simulink model "Auto_microgrid_forecasting_020822"  (R2020a)
settings: Solver=VariableStepAuto  StartTime=0.0  StopTime=50  MaxStep=1e-4  RelTol=1e-3
PreLoadFcn:
  | %run('FC_microgrid_param.m')
  | %load('gen_grid_init.mat')
InitFcn:
  | %load myisoModel_init;
  | run('FC_microgrid_param.m')
  | tic
  | run('CARTinitFcn.m')
  | %caseNo = 2;
  | 
  | %if (caseNo == 1)
  | %set_param(['Isolated_grid_paper_model_022521/SignalGen'], 'ActiveScenario', 'PStep222kW');
  | %else
  | %set_param(['Isolated_grid_paper_model_022521/SignalGen'], 'ActiveScenario', 'QStep222kVAr');
  | 
  | %end;
StopFcn:
  | toc
undefined symbols (not defined in the file or in its folder): breakpoints1, breakpoints2, cc_kp, cp_table_data, ctrl, D1, Delta, DiscIntNeverNeededParam, DT, FC_BESS, FC_PV_FirstSolar, find_system, Fnom, gcbh, libFC_BESS, libFC_PV, LowerLimit, magnitude, oversize, pll_ki, pll_kp, pq_ts, SOC_target, sps_rtmsupport, timer, Ts, ts, Ts_APC, Ts_Control, Ts_Power, UpperLimit
libraries: powerlib x151, simulink x100, powerlib_extras x100, powerlib_meascontrol x91, eePowerMeasurement x26, pi_ctrl x16, simulink_extras x12, sps_avr x7, eeGeneralControl x5, spsDieselMotorModel x3, libFSArray x2, SignalEditorBlockLib x2
(part 3 of 14)

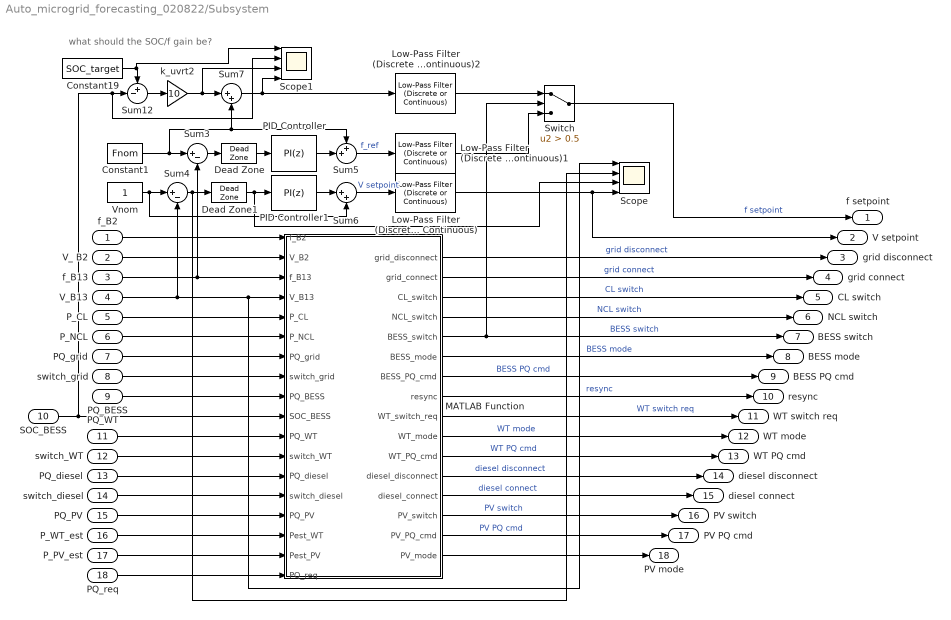
== system Auto_microgrid_forecasting_020822/Subsystem ==
  note: what should the SOC/f gain be?
  f_B2 : Inport
  V_ B2 : Inport  Port=2
  f_B13 : Inport  Port=3
  V_B13 : Inport  Port=4
  P_CL : Inport  Port=5
  P_NCL : Inport  Port=6
  PQ_grid : Inport  Port=7
  switch_grid : Inport  Port=8
  PQ_BESS : Inport  Port=9
  SOC_BESS : Inport  Port=10
  PQ_WT : Inport  Port=11
  switch_WT : Inport  Port=12
  PQ_diesel : Inport  Port=13
  switch_diesel : Inport  Port=14
  PQ_PV : Inport  Port=15
  P_WT_est : Inport  Port=16
  P_PV_est : Inport  Port=17
  PQ_req : Inport  Port=18
  Constant1 : Constant  Value=Fnom  SampleTime=-1
  Constant19 : Constant  Value=SOC_target  SampleTime=-1
  Dead Zone : DeadZone  LowerValue=-0.036  UpperValue=0.036  SaturateOnIntegerOverflow=on
  Dead Zone1 : DeadZone  LowerValue=-0.005  UpperValue=0.005  SaturateOnIntegerOverflow=on
  Low-Pass Filter (Discrete or Continuous) : eeGeneralControl/Low-Pass Filter (Discrete or Continuous)  K=1  T=0.2  B=inf  A=-inf  init_option=Inherited from block input  x0=0  Ts=-1
  Low-Pass Filter (Discrete or Continuous)1 : eeGeneralControl/Low-Pass Filter (Discrete or Continuous)  K=1  T=0.2  B=inf  A=-inf  init_option=Inherited from block input  x0=0  Ts=-1
  Low-Pass Filter (Discrete or Continuous)2 : eeGeneralControl/Low-Pass Filter (Discrete or Continuous)  K=1  T=0.2  B=inf  A=-inf  init_option=Inherited from block input  x0=0  Ts=-1
  MATLAB Function : MATLAB Function  TreatAsAtomicUnit=on
  PID Controller : simulink/Continuous/PID Controller  Controller=PI  Form=Parallel  TimeDomain=Discrete-time  UseExternalTs=off  SampleTime=-1  IntegratorMethod=Forward Euler  FilterMethod=Forward Euler  ControllerParametersSource=internal  P=1  I=1/10  D=0  UseFilter=on  N=100  TunerSelectOption=Transfer Function Based (PID Tuner App)  InitialConditionSource=internal  InitialConditionForIntegrator=0  InitialConditionForFilter=0  DifferentiatorICPrevScaledInput=0  ExternalReset=none  TrackingMode=off  Kt=1  LimitOutput=off  UpperSaturationLimit=inf  LowerSaturationLimit=-inf  LinearizeAsGain=on  AntiWindupMode=none  Kb=1  POutMin=[]  POutMax=[]  IOutMin=[]  IOutMax=[]  DOutMin=[]  DOutMax=[]  NOutMin=[]  NOutMax=[]  SumOutMin=[]  SumOutMax=[]  SaturationOutMin=[]  SaturationOutMax=[]  PParamMin=[]  PParamMax=[]  IParamMin=[]  IParamMax=[]  DParamMin=[]  DParamMax=[]  NParamMin=[]  NParamMax=[]  KbParamMin=[]  KbParamMax=[]  KtParamMin=[]  KtParamMax=[]  KbOutMin=[]  KbOutMax=[]  KtOutMin=[]  KtOutMax=[]  IntegratorOutMin=[]  IntegratorOutMax=[]  FilterOutMin=[]  FilterOutMax=[]  SumI1OutMin=[]  SumI1OutMax=[]  SumI2OutMin=[]  SumI2OutMax=[]  SumI3OutMin=[]  SumI3OutMax=[]  SumI4OutMin=[]  SumI4OutMax=[]  SumDOutMin=[]  SumDOutMax=[]  DifferentiatorOutMin=[]  DifferentiatorOutMax=[]  FilterDiffOutCoefMin=[]  FilterDiffOutCoefMax=[]  ReciprocalOutMin=[]  ReciprocalOutMax=[]  SumDenOutMin=[]  SumDenOutMax=[]  SumNumOutMin=[]  SumNumOutMax=[]  DivideOutMin=[]  DivideOutMax=[]  UdiffTsProdOutMin=[]  UdiffTsProdOutMax=[]  NTsProdOutMin=[]  NTsProdOutMax=[]  UintegralTsProdOutMin=[]  UintegralTsProdOutMax=[]  UngainTsProdOutMin=[]  UngainTsProdOutMax=[]  IntegratorContinuousStateAttributes=''  IntegratorStateMustResolveToSignalObject=off  IntegratorRTWStateStorageClass=Auto  FilterContinuousStateAttributes=''  FilterStateMustResolveToSignalObject=off  FilterRTWStateStorageClass=Auto  ParallelPVariant=InternalParameters  IdealPVariant=Disabled  IVariant=InternalParameters  DVariant=Disabled  IntegratorVariant=Discrete  SatVariant=Disabled  AWVariant=Passthrough  PCopyVariant=Disabled  TRVariant=Disabled  FdbkBlocksVariant=Forward  IdealPFdbkVariant=Disabled  SatFdbkVariant=Disabled  DerivativeFilterVariant=Disabled  NVariant=Disabled  NCopyVariant=Disabled_SignalSpec  FilterICVariant=Disabled  IntegratorICVariant=InternalICs  ExternalResetVariant=Disabled  TRSumVariant=Passthrough  SumFdbkVariant=Disabled  SumVariant=Sum_PI  TsampFilterVariant=InternalTs  TsampNgainVariant=Passthrough  TsampIntegralVariant=Passthrough
  PID Controller1 : simulink/Continuous/PID Controller  Controller=PI  Form=Parallel  TimeDomain=Discrete-time  UseExternalTs=off  SampleTime=-1  IntegratorMethod=Forward Euler  FilterMethod=Forward Euler  ControllerParametersSource=internal  P=1  I=1/10  D=0  UseFilter=on  N=100  TunerSelectOption=Transfer Function Based (PID Tuner App)  InitialConditionSource=internal  InitialConditionForIntegrator=0  InitialConditionForFilter=0  DifferentiatorICPrevScaledInput=0  ExternalReset=none  TrackingMode=off  Kt=1  LimitOutput=off  UpperSaturationLimit=inf  LowerSaturationLimit=-inf  LinearizeAsGain=on  AntiWindupMode=none  Kb=1  POutMin=[]  POutMax=[]  IOutMin=[]  IOutMax=[]  DOutMin=[]  DOutMax=[]  NOutMin=[]  NOutMax=[]  SumOutMin=[]  SumOutMax=[]  SaturationOutMin=[]  SaturationOutMax=[]  PParamMin=[]  PParamMax=[]  IParamMin=[]  IParamMax=[]  DParamMin=[]  DParamMax=[]  NParamMin=[]  NParamMax=[]  KbParamMin=[]  KbParamMax=[]  KtParamMin=[]  KtParamMax=[]  KbOutMin=[]  KbOutMax=[]  KtOutMin=[]  KtOutMax=[]  IntegratorOutMin=[]  IntegratorOutMax=[]  FilterOutMin=[]  FilterOutMax=[]  SumI1OutMin=[]  SumI1OutMax=[]  SumI2OutMin=[]  SumI2OutMax=[]  SumI3OutMin=[]  SumI3OutMax=[]  SumI4OutMin=[]  SumI4OutMax=[]  SumDOutMin=[]  SumDOutMax=[]  DifferentiatorOutMin=[]  DifferentiatorOutMax=[]  FilterDiffOutCoefMin=[]  FilterDiffOutCoefMax=[]  ReciprocalOutMin=[]  ReciprocalOutMax=[]  SumDenOutMin=[]  SumDenOutMax=[]  SumNumOutMin=[]  SumNumOutMax=[]  DivideOutMin=[]  DivideOutMax=[]  UdiffTsProdOutMin=[]  UdiffTsProdOutMax=[]  NTsProdOutMin=[]  NTsProdOutMax=[]  UintegralTsProdOutMin=[]  UintegralTsProdOutMax=[]  UngainTsProdOutMin=[]  UngainTsProdOutMax=[]  IntegratorContinuousStateAttributes=''  IntegratorStateMustResolveToSignalObject=off  IntegratorRTWStateStorageClass=Auto  FilterContinuousStateAttributes=''  FilterStateMustResolveToSignalObject=off  FilterRTWStateStorageClass=Auto  ParallelPVariant=InternalParameters  IdealPVariant=Disabled  IVariant=InternalParameters  DVariant=Disabled  IntegratorVariant=Discrete  SatVariant=Disabled  AWVariant=Passthrough  PCopyVariant=Disabled  TRVariant=Disabled  FdbkBlocksVariant=Forward  IdealPFdbkVariant=Disabled  SatFdbkVariant=Disabled  DerivativeFilterVariant=Disabled  NVariant=Disabled  NCopyVariant=Disabled_SignalSpec  FilterICVariant=Disabled  IntegratorICVariant=InternalICs  ExternalResetVariant=Disabled  TRSumVariant=Passthrough  SumFdbkVariant=Disabled  SumVariant=Sum_PI  TsampFilterVariant=InternalTs  TsampNgainVariant=Passthrough  TsampIntegralVariant=Passthrough
  Scope : Scope  NumInputPorts=4
  Scope1 : Scope  NumInputPorts=4
  Sum12 : Sum  Inputs=+-|
  Sum3 : Sum  Inputs=|+-
  Sum4 : Sum  Inputs=|+-
  Sum5 : Sum  Inputs=++|
  Sum6 : Sum  Inputs=|++
  Sum7 : Sum  Inputs=|++
  Switch : Switch  Criteria=u2 > Threshold  Threshold=0.5
  Vnom : Constant  SampleTime=-1
  k_uvrt2 : Gain  Gain=10
  f setpoint : Outport
  V setpoint : Outport  Port=2
  grid disconnect : Outport  Port=3
  grid connect : Outport  Port=4
  CL switch : Outport  Port=5
  NCL switch : Outport  Port=6
  BESS switch : Outport  Port=7
  BESS mode : Outport  Port=8
  BESS PQ cmd : Outport  Port=9
  resync : Outport  Port=10
  WT switch req : Outport  Port=11
  WT mode : Outport  Port=12
  WT PQ cmd : Outport  Port=13
  diesel disconnect : Outport  Port=14
  diesel connect : Outport  Port=15
  PV switch : Outport  Port=16
  PV PQ cmd : Outport  Port=17
  PV mode : Outport  Port=18
  wires:
  Vnom/1 -> Sum6/2, Sum4/1
  MATLAB Function/15(PV_PQ_cmd) -> PV PQ cmd/1  "PV PQ cmd"
  Constant1/1 -> Sum5/1, Sum7/2, Sum3/1
  switch_diesel/1 -> MATLAB Function/14(switch_diesel)
  P_PV_est/1 -> MATLAB Function/17(Pest_PV)
  Sum4/1 -> Scope/2, Dead Zone1/1
  MATLAB Function/6(BESS_mode) -> BESS mode/1  "BESS mode"
  PQ_WT/1 -> MATLAB Function/11(PQ_WT)
  P_CL/1 -> MATLAB Function/5(P_CL)
  PID Controller/1 -> Sum5/2
  Constant19/1 -> Scope1/1, Sum12/1
  MATLAB Function/5(BESS_switch) -> BESS switch/1, Switch/2  "BESS switch"
  Dead Zone/1 -> PID Controller/1
  SOC_BESS/1 -> MATLAB Function/10(SOC_BESS), Scope1/2, Sum12/2
  Sum3/1 -> Dead Zone/1
  Switch/1 -> f setpoint/1  "f setpoint"
  PQ_BESS/1 -> MATLAB Function/9(PQ_BESS)
  Dead Zone1/1 -> Scope/3, PID Controller1/1
  PID Controller1/1 -> Sum6/1
  Sum12/1 -> k_uvrt2/1
  MATLAB Function/1(grid_disconnect) -> grid disconnect/1  "grid disconnect"
  MATLAB Function/12(diesel_disconnect) -> diesel disconnect/1  "diesel disconnect"
  switch_grid/1 -> MATLAB Function/8(switch_grid)
  P_NCL/1 -> MATLAB Function/6(P_NCL)
  k_uvrt2/1 -> Scope1/3, Sum7/1
  Sum5/1 -> Low-Pass Filter (Discrete or Continuous)1/1  "f_ref"
  switch_WT/1 -> MATLAB Function/12(switch_WT)
  Sum7/1 -> Scope1/4, Low-Pass Filter (Discrete or Continuous)2/1
  MATLAB Function/4(NCL_switch) -> NCL switch/1  "NCL switch"
  MATLAB Function/7(BESS_PQ_cmd) -> BESS PQ cmd/1  "BESS PQ cmd"
  PQ_PV/1 -> MATLAB Function/15(PQ_PV)
  Sum6/1 -> Low-Pass Filter (Discrete or Continuous)/1  "V setpoint"
  V_ B2/1 -> MATLAB Function/2(V_B2)
  MATLAB Function/2(grid_connect) -> grid connect/1  "grid connect"
  P_WT_est/1 -> MATLAB Function/16(Pest_WT)
  PQ_diesel/1 -> MATLAB Function/13(PQ_diesel)
  MATLAB Function/11(WT_PQ_cmd) -> WT PQ cmd/1  "WT PQ cmd"
  PQ_grid/1 -> MATLAB Function/7(PQ_grid)
  MATLAB Function/8(resync) -> resync/1  "resync"
  MATLAB Function/10(WT_mode) -> WT mode/1  "WT mode"
  MATLAB Function/3(CL_switch) -> CL switch/1  "CL switch"
  MATLAB Function/14(PV_switch) -> PV switch/1  "PV switch"
  MATLAB Function/9(WT_switch_req) -> WT switch req/1  "WT switch req"
  MATLAB Function/13(diesel_connect) -> diesel connect/1  "diesel connect"
  V_B13/1 -> Scope/1, MATLAB Function/4(V_B13), Sum4/2
  Low-Pass Filter (Discrete or Continuous)/1 -> Scope/4, V setpoint/1
  Low-Pass Filter (Discrete or Continuous)1/1 -> Switch/3
  Low-Pass Filter (Discrete or Continuous)2/1 -> Switch/1
  MATLAB Function/16(PV_mode) -> PV mode/1
  f_B2/1 -> MATLAB Function/1(f_B2)
  f_B13/1 -> MATLAB Function/3(f_B13), Sum3/2
  PQ_req/1 -> MATLAB Function/18(PQ_req)

== system Auto_microgrid_forecasting_020822/Subsystem1 ==
  freq : Inport
  Voltage : Inport  Port=2
  AND : Logic  Inputs=3  IconShape=distinctive  AllPortsSameDT=off  OutDataTypeStr=boolean
  Bus Selector : BusSelector  OutputSignals=NCL switch
  Compare To Constant{1..4} (4 alike) : simulink/Logic and Bit Operations/Compare To Constant  relop=>  const=0.1  OutDataTypeStr=boolean
  Constant : Constant  Value=60
  Constant1 : Constant
  Data Type Conversion{,1..3} (4 alike) : DataTypeConversion
  Digital Clock : DigitalClock  SampleTime=Ts
  Digital Clock1 : DigitalClock  SampleTime=Ts
  Discrete-Time Integrator{1..4} (4 alike) : DiscreteIntegrator  ExternalReset=falling  SampleTime=Ts  ICPrevOutput=DiscIntNeverNeededParam  ICPrevScaledInput=DiscIntNeverNeededParam
  Gain9 : Gain  Gain=1/13200*sqrt(3/2)
  NOR : Logic  Operator=NOR  IconShape=distinctive  AllPortsSameDT=off  OutDataTypeStr=boolean
  NOR1 : Logic  Operator=NOR  IconShape=distinctive  AllPortsSameDT=off  OutDataTypeStr=boolean
  Scope : Scope  NumInputPorts=2
  Switch : Switch  Criteria=u2 > Threshold  Threshold=1
  Switch1 : Switch  Criteria=u2 > Threshold  Threshold=1
  umax : simulink/Logic and Bit Operations/Compare To Constant  relop=<=  const=58  OutDataTypeStr=boolean
  umax1 : simulink/Logic and Bit Operations/Compare To Constant  relop=>=  const=61.8  OutDataTypeStr=boolean
  umax2 : simulink/Logic and Bit Operations/Compare To Constant  relop=<=  const=0  OutDataTypeStr=boolean
  umax3 : simulink/Logic and Bit Operations/Compare To Constant  relop=>=  const=1.3  OutDataTypeStr=boolean
  control : Outport
  wires:
  Data Type Conversion1/1 -> Discrete-Time Integrator1/2, Discrete-Time Integrator1/1
  Compare To Constant1/1 -> NOR/2
  Discrete-Time Integrator2/1 -> Compare To Constant2/1
  umax1/1 -> Data Type Conversion1/1
  Data Type Conversion/1 -> Discrete-Time Integrator2/2, Discrete-Time Integrator2/1
  umax/1 -> Data Type Conversion/1
  Discrete-Time Integrator1/1 -> Compare To Constant1/1
  Compare To Constant2/1 -> NOR/1
  NOR/1 -> Scope/1, AND/1
  Compare To Constant4/1 -> NOR1/1
  Discrete-Time Integrator3/1 -> Compare To Constant3/1
  umax2/1 -> Data Type Conversion2/1
  umax3/1 -> Data Type Conversion3/1
  Data Type Conversion3/1 -> Discrete-Time Integrator3/2, Discrete-Time Integrator3/1
  Data Type Conversion2/1 -> Discrete-Time Integrator4/2, Discrete-Time Integrator4/1
  Discrete-Time Integrator4/1 -> Compare To Constant4/1
  Compare To Constant3/1 -> NOR1/2
  NOR1/1 -> Scope/2, AND/2
  AND/1 -> control/1
  freq/1 -> Switch/1
  Switch/1 -> umax1/1, umax/1
  Constant/1 -> Switch/3
  Digital Clock/1 -> Switch/2
  Voltage/1 -> Gain9/1
  Digital Clock1/1 -> Switch1/2
  Constant1/1 -> Switch1/3
  Switch1/1 -> umax3/1, umax2/1
  Gain9/1 -> Switch1/1  "V [pu]"
  [MGCC_cmd] -> Bus Selector/1
  Bus Selector/1 -> AND/3  "<NCL switch>"

== system Auto_microgrid_forecasting_020822/Subsystem2 ==
  freq : Inport
  Voltage : Inport  Port=2
  AND : Logic  Inputs=3  IconShape=distinctive  AllPortsSameDT=off  OutDataTypeStr=boolean
  Bus Selector : BusSelector  OutputSignals=CL switch
  Compare To Constant{1..4} (4 alike) : simulink/Logic and Bit Operations/Compare To Constant  relop=>  const=0.1  OutDataTypeStr=boolean
  Constant : Constant  Value=60
  Constant1 : Constant
  Data Type Conversion{,1..3} (4 alike) : DataTypeConversion
  Digital Clock : DigitalClock  SampleTime=Ts
  Digital Clock1 : DigitalClock  SampleTime=Ts
  Discrete-Time Integrator{1..4} (4 alike) : DiscreteIntegrator  ExternalReset=falling  SampleTime=Ts  ICPrevOutput=DiscIntNeverNeededParam  ICPrevScaledInput=DiscIntNeverNeededParam
  Gain9 : Gain  Gain=1/13200*sqrt(3/2)
  NOR : Logic  Operator=NOR  IconShape=distinctive  AllPortsSameDT=off  OutDataTypeStr=boolean
  NOR1 : Logic  Operator=NOR  IconShape=distinctive  AllPortsSameDT=off  OutDataTypeStr=boolean
  Scope : Scope  NumInputPorts=2
  Switch : Switch  Criteria=u2 > Threshold  Threshold=1
  Switch1 : Switch  Criteria=u2 > Threshold  Threshold=1
  umax : simulink/Logic and Bit Operations/Compare To Constant  relop=<=  const=57  OutDataTypeStr=boolean
  umax1 : simulink/Logic and Bit Operations/Compare To Constant  relop=>=  const=63  OutDataTypeStr=boolean
  umax2 : simulink/Logic and Bit Operations/Compare To Constant  relop=<=  const=0  OutDataTypeStr=boolean
  umax3 : simulink/Logic and Bit Operations/Compare To Constant  relop=>=  const=1.5  OutDataTypeStr=boolean
  control : Outport
  wires:
  Data Type Conversion1/1 -> Discrete-Time Integrator1/2, Discrete-Time Integrator1/1
  Compare To Constant1/1 -> NOR/2
  Discrete-Time Integrator2/1 -> Compare To Constant2/1
  umax1/1 -> Data Type Conversion1/1
  Data Type Conversion/1 -> Discrete-Time Integrator2/2, Discrete-Time Integrator2/1
  umax/1 -> Data Type Conversion/1
  Discrete-Time Integrator1/1 -> Compare To Constant1/1
  Compare To Constant2/1 -> NOR/1
  NOR/1 -> Scope/1, AND/1
  Compare To Constant4/1 -> NOR1/1
  Discrete-Time Integrator3/1 -> Compare To Constant3/1
  umax2/1 -> Data Type Conversion2/1
  umax3/1 -> Data Type Conversion3/1
  Data Type Conversion3/1 -> Discrete-Time Integrator3/2, Discrete-Time Integrator3/1
  Data Type Conversion2/1 -> Discrete-Time Integrator4/2, Discrete-Time Integrator4/1
  Discrete-Time Integrator4/1 -> Compare To Constant4/1
  Compare To Constant3/1 -> NOR1/2
  NOR1/1 -> Scope/2, AND/2
  AND/1 -> control/1
  Constant/1 -> Switch/3
  Voltage/1 -> Gain9/1
  Digital Clock/1 -> Switch/2
  Switch/1 -> umax1/1, umax/1
  freq/1 -> Switch/1
  Digital Clock1/1 -> Switch1/2
  Constant1/1 -> Switch1/3
  Switch1/1 -> umax3/1, umax2/1
  Gain9/1 -> Switch1/1  "V [pu]"
  Bus Selector/1 -> AND/3  "<CL switch>"
  [MGCC_cmd] -> Bus Selector/1

== system Auto_microgrid_forecasting_020822/Subsystem4 ==
  Generator Bus : Subsystem
  a : PMIOPort  Side=Left
  b : PMIOPort  Port=2  Side=Left
  c : PMIOPort  Port=3  Side=Left
  Conn6 : PMIOPort  Port=4  Side=Right
  Conn4 : PMIOPort  Port=5  Side=Right
  Conn5 : PMIOPort  Port=6  Side=Right
  connections:
  Generator Bus/RConn2 -- b/RConn1
  Conn4/RConn1 -- Generator Bus/LConn1
  Conn5/RConn1 -- Generator Bus/LConn2
  Conn6/RConn1 -- Generator Bus/LConn3
  c/RConn1 -- Generator Bus/RConn3
  a/RConn1 -- Generator Bus/RConn1

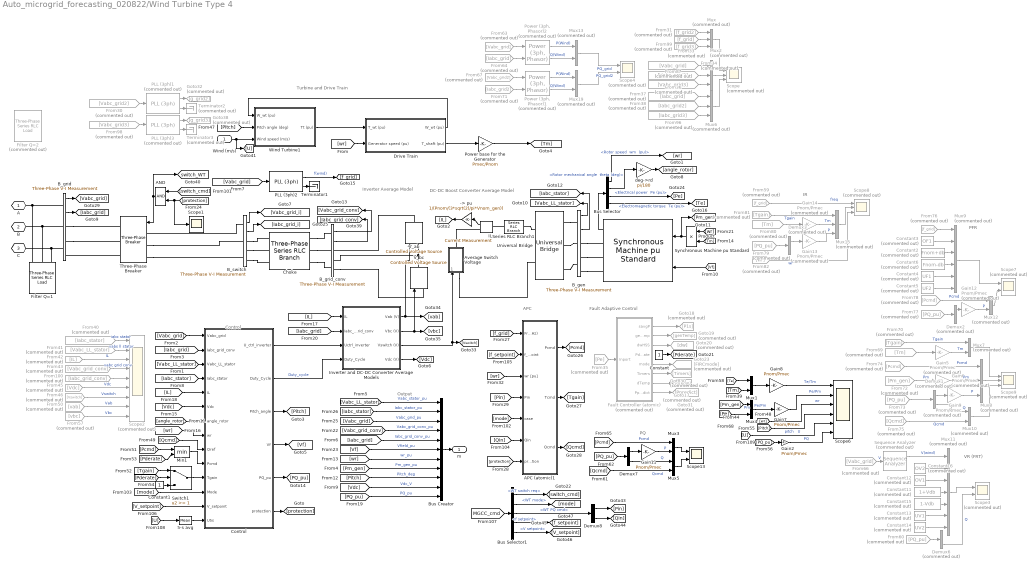
== system Auto_microgrid_forecasting_020822/Wind Turbine Type 4 ==
  note: Control
  note: Turbine and Drive Train
  note: Inverter
      | Average Model
  note: DC-DC Boost Converter
      | Average Model
  note: Fault Adaptive Control
  note: PFR
  note: IR
  note: PQ
  note: APC
  note: Output
  note: VR (FRT)
  "Wind (m/s) " : Inport
  -> pu : Gain  Gain=1/(Pnom/(3*sqrt(2)/pi*Vnom_gen))  SaturateOnIntegerOverflow=on  OutDataTypeStr=Inherit: Same as input  ParamDataTypeStr=Inherit: Same as input
  5-s avg : powerlib_meascontrol/Measurements/Mean  Freq=5  Vinit=15  Ts=Ts
  AND : Logic  IconShape=distinctive  AllPortsSameDT=off  OutDataTypeStr=boolean
  APC (atomic)1 : Subsystem  TreatAsAtomicUnit=on  SystemSampleTime=0.01
  Average Switch Voltage : Subsystem
  B_gen : powerlib/Measurements/Three-Phase V-I Measurement  VoltageMeasurement=phase-to-phase  SetLabelV=off  LabelV=Vabc  Vpu=on  VpuLL=off  CurrentMeasurement=yes  SetLabelI=off  LabelI=Iabc  Ipu=on  Pbase=Pnom  Vbase=Vnom_gen  OutputType=Complex  PhasorSimulation=off  PSBequivalent=0
      settings: SourceProductBaseCode=MT,PS
  B_grid : powerlib/Measurements/Three-Phase V-I Measurement  VoltageMeasurement=phase-to-ground  SetLabelV=off  LabelV=Vabc  Vpu=on  VpuLL=off  CurrentMeasurement=yes  SetLabelI=off  LabelI=Iabc  Ipu=on  Pbase=Pnom  Vbase=Vnom  OutputType=Complex  PhasorSimulation=off  PSBequivalent=0
      settings: SourceProductBaseCode=MT,PS
  B_grid_conv : powerlib/Measurements/Three-Phase V-I Measurement  VoltageMeasurement=phase-to-ground  SetLabelV=off  LabelV=Vabc  Vpu=on  VpuLL=off  CurrentMeasurement=yes  SetLabelI=off  LabelI=Iabc  Ipu=on  Pbase=Pnom  Vbase=Vnom  OutputType=Complex  PhasorSimulation=off  PSBequivalent=0
      settings: SourceProductBaseCode=MT,PS
  B_switch : powerlib/Measurements/Three-Phase V-I Measurement  VoltageMeasurement=phase-to-ground  SetLabelV=off  LabelV=Vabc  Vpu=on  VpuLL=off  CurrentMeasurement=yes  SetLabelI=off  LabelI=Iabc  Ipu=on  Pbase=Pnom  Vbase=Vnom  OutputType=Complex  PhasorSimulation=off  PSBequivalent=0
      settings: SourceProductBaseCode=MT,PS
  Bus Creator : BusCreator  Inputs=11
  Bus Selector : BusSelector  OutputSignals="Mechanical.Rotor speed  wm  (pu),Mechanical.Rotor mechanical angle  theta (deg),Mechanical.Electrical power  Pe (pu),Mechanical.Electromagnetic torque  Te (pu)"
  Bus Selector1 : BusSelector  OutputSignals=WT switch req,WT mode,WT PQ cmd,f setpoint,V setpoint
  "Choke " : powerlib/Elements/Three-Phase Series RLC Branch  LConnTagsString=A|B|C  RConnTagsString=A|B|C  BranchType=RL  Resistance=R_RL*Vnom^2/Pnom  Inductance=L_RL*Vnom^2/Pnom/(2*pi*Fnom)  Capacitance=[]  Measurements=None
      settings: SourceProductBaseCode=MT,PS
  Constant : Constant
  Constant1 : Constant
  Constant11 : Constant  Commented=on  Value=1+Vdb
  Constant12 : Constant  Commented=on  Value=OV1
  Constant13 : Constant  Commented=on  Value=UV1
  Constant14 : Constant  Commented=on  Value=UV2
  Constant15 : Constant  Commented=on  Value=1-Vdb
  Constant16 : Constant  Commented=on  Value=OV2
  Constant2 : Constant  Commented=on  Value=Fnom+db
  Constant3 : Constant  Commented=on  Value=OF1
  Constant4 : Constant  Commented=on  Value=UF1
  Constant5 : Constant  Commented=on  Value=UF2
  Constant6 : Constant  Commented=on  Value=Fnom-db
  Control : Subsystem
  Demux{1..3,6} (4 alike) : Demux  Commented=on  Outputs=2
  Demux7 : Demux  Outputs=2
  Demux8 : Demux  Outputs=2
  Drive Train : Subsystem  mask(Wind Turbine shaft){H_WT=H_WT/10, Ksh=Ksh, D_mutual=D_mutual, wbase=2*pi*Fnom/p, w_wt0=w_wt0, torque0=torque0, Ts=Ts}
      mask prompts: H_WT "Wind turbine inertia constant H (s):"; Ksh "Shaft spring constant (pu of nominal mechanical torque/rad):"; D_mutual "Shaft mutual damping (pu of nominal mechanical torque/pu dw):"; wbase "Shaft base speed (rad/s):"; w_wt0 "Turbine initial speed (pu of base speed):"; torque0 "Initial output torque (pu of nominal mechanical torque):"; Ts "Sample time (s):"
      mask help:
      | This block implements a wind turbine drive train model. All shaft parameters are referred to high-speed shaft (generator shaft).
      |
      | The first input is the wind turbine torque in per unit (pu) based on the nominal power of the turbine and the base speed of the generator. The second input is the generator speed in pu based on the base speed of the generator.
      |
      | The outputs are:
      | 1- the transmitted torque of the shaft in pu based on the nominal power of the turbine and the base speed of the generator.
      | 2- the wind turbine speed in pu of the base speed of the generator.
  "Fault Controller (atomic) " : Subsystem  Commented=on  TreatAsAtomicUnit=on  SystemSampleTime=Ts_APC
  Filter Q=1 : powerlib/Elements/Three-Phase Series RLC Load  LConnTagsString=A|B|C  Configuration=Y (grounded)  NominalVoltage=Vnom  Vabc=[1e3 1e3 1e3]  Vabcp=[1e3 1e3 1e3]  NominalFrequency=Fnom  UnbalancedPower=off  ActivePower=100  InductivePower=100  CapacitivePower=100  Pabc=[10e3 9e3 11e3]  QLabc=[100 90 110]  QCabc=[100 90 110]  Pabcp=[10e3 9e3 11e3]  QLabcp=[100 90 110]  QCabcp=[100 90 110]  Measurements=None  LoadType=constant Z
      settings: SourceProductBaseCode=MT,PS
  Filter Q=2 : powerlib/Elements/Three-Phase Series RLC Load  Commented=on  LConnTagsString=A|B|C  Configuration=Y (grounded)  NominalVoltage=Vnom  Vabc=[1e3 1e3 1e3]  Vabcp=[1e3 1e3 1e3]  NominalFrequency=Fnom  UnbalancedPower=off  ActivePower=C_var_filter/Q_filter  InductivePower=0  CapacitivePower=C_var_filter  Pabc=[10e3 9e3 11e3]  QLabc=[100 90 110]  QCabc=[100 90 110]  Pabcp=[10e3 9e3 11e3]  QLabcp=[100 90 110]  QCabcp=[100 90 110]  Measurements=None  LoadType=constant Z
      settings: SourceProductBaseCode=MT,PS
  From100 : From  Commented=on  GotoTag=Iabc_grid_conv
  From30 : From  Commented=on  GotoTag=Vabc_grid2
  From31 : From  Commented=on  GotoTag=f_grid2
  From33 : From  Commented=on  GotoTag=f_grid
  From34 : From  Commented=on  GotoTag=Vabc_grid
  From35 : From  Commented=on  GotoTag=Pe
  From36 : From  Commented=on  GotoTag=Vabc_grid2
  From37 : From  Commented=on  GotoTag=Iabc_grid
  From38 : From  Commented=on  GotoTag=Iabc_grid2
  From40 : From  Commented=on  GotoTag=Iabc_stator
  From41 : From  Commented=on  GotoTag=Vabc_LL_stator
  From42 : From  Commented=on  GotoTag=IL
  From43 : From  Commented=on  GotoTag=Vabc_grid_conv
  From45 : From  Commented=on  GotoTag=Vdc
  From46 : From  Commented=on  GotoTag=Vswitch
  From50 : From  Commented=on  GotoTag=vab
  From57 : From  Commented=on  GotoTag=vbc
  From59 : From  Commented=on  GotoTag=f_grid
  From{60,73,77,79} (4 alike) : From  Commented=on  GotoTag=PQ_pu
  From63 : From  Commented=on  GotoTag=Vabc_grid
  From64 : From  Commented=on  GotoTag=Iabc_grid
  From66 : From  Commented=on  GotoTag=Vabc_grid
      settings: CloseFcn=tagdialog Close
  From67 : From  Commented=on  GotoTag=Vabc_grid2
  From69 : From  Commented=on  GotoTag=Tm
  From70 : From  Commented=on  GotoTag=Tgain
  From71 : From  Commented=on  GotoTag=Iabc_grid2
  From72 : From  Commented=on  GotoTag=Pm_gen
  From74 : From  Commented=on  GotoTag=Pcmd
  From75 : From  Commented=on  GotoTag=Qcmd
  From76 : From  Commented=on  GotoTag=f_grid
  From78 : From  Commented=on  GotoTag=Pcmd
  From80 : From  Commented=on  GotoTag=Tm
  From81 : From  Commented=on  GotoTag=Tgain
  From82 : From  Commented=on  GotoTag=wr
  From87 : From  Commented=on  GotoTag=Vabc_grid3
  From96 : From  Commented=on  GotoTag=Iabc_grid3
  From98 : From  Commented=on  GotoTag=Vabc_grid3
  From99 : From  Commented=on  GotoTag=f_grid3
  Gain{2,7..8,11} (4 alike) : Gain  Gain=Pnom/Pmec
  Gain{5..6,9,12..14} (6 alike) : Gain  Commented=on  Gain=Pnom/Pmec
  Goto17 : Goto  Commented=on  GotoTag=dTemp
  Goto18 : Goto  Commented=on  GotoTag=P1s
  Goto19 : Goto  Commented=on  GotoTag=genTemp
  Goto20 : Goto  Commented=on  GotoTag=dw
  Goto23 : Goto  Commented=on  GotoTag=FIRCmode
  Goto30 : Goto  Commented=on  GotoTag=Timers
  Goto31 : Goto  Commented=on  GotoTag=Ppredict
  Goto32 : Goto  Commented=on  GotoTag=g_grid2
  Goto38 : Goto  Commented=on  GotoTag=g_grid3
  IL : powerlib/Measurements/Current Measurement  PhasorSimulation=off  OutputType=Complex  PSBequivalent=0
      settings: SourceProductBaseCode=MT,PS
  Inverter and DC-DC Converter Average Models : Subsystem
  Min1 : MinMax  Inputs=2
  Mux{,2,6,8,15} (5 alike) : Mux  Commented=on  Inputs=3
  Mux{1,3..5} (4 alike) : Mux  Inputs=2
  Mux{7,10,12..13,19} (5 alike) : Mux  Commented=on  Inputs=2
  Mux11 : Mux  Commented=on  Inputs=7
  Mux9 : Mux  Commented=on  Inputs=6
  PLL (3ph)1 : powerlib_meascontrol/PLL/PLL (3ph)  Commented=on  Fmin=45  Par_Init=[0, 60]  ParK=[180, 3200, 1]  TcD=1e-4  MaxRateChangeFreq=12  FilterCutOffFreq=25  Ts=Ts  AGC=on
  PLL (3ph)2 : powerlib_meascontrol/PLL/PLL (3ph)  Fmin=45  Par_Init=[0, 60]  ParK=[180, 3200, 1]  TcD=1e-4  MaxRateChangeFreq=12  FilterCutOffFreq=25  Ts=Ts  AGC=on
  PLL (3ph)3 : powerlib_meascontrol/PLL/PLL (3ph)  Commented=on  Fmin=45  Par_Init=[0, 60]  ParK=[180, 3200, 1]  TcD=1e-4  MaxRateChangeFreq=12  FilterCutOffFreq=25  Ts=Ts  AGC=on
  "Power (3ph, Phasor)1" : powerlib_meascontrol/Measurements/Power (3ph, Phasor)  Commented=on
      settings: SourceProductBaseCode=PS
  "Power (3ph, Phasor)2" : powerlib_meascontrol/Measurements/Power (3ph, Phasor)  Commented=on
      settings: SourceProductBaseCode=PS
  Power base for the Generator : Gain  Gain=Pmec/Pnom  SaturateOnIntegerOverflow=on  OutDataTypeStr=Inherit: Same as input  ParamDataTypeStr=Inherit: Same as input
  Product : Product  RndMeth=Zero
  Scope : Scope  Commented=on  NumInputPorts=3
  Scope1 : Scope
  Scope13 : Scope  NumInputPorts=2
  Scope2 : Scope  Commented=on  NumInputPorts=9
  Scope3 : Scope  Commented=on  NumInputPorts=2
  Scope4 : Scope  Commented=on  NumInputPorts=2
  Scope6 : Scope  NumInputPorts=6
  Scope7 : Scope  Commented=on  NumInputPorts=2
  Scope8 : Scope  Commented=on  NumInputPorts=3
  Scope9 : Scope  Commented=on  NumInputPorts=3
  Sequence Analyzer : powerlib_meascontrol/Measurements/Sequence Analyzer  Commented=on  Freq=60  n=1  seq=Positive  InInit=[1, 0]  Ts=Ts
      settings: SourceProductBaseCode=PS
  Series RLC Branch1 : powerlib/Elements/Series RLC Branch  LConnTagsString=__new0  RConnTagsString=__new0  BranchType=RL  Resistance=R_Boost  Inductance=L_Boost  SetiL0=off  InitialCurrent=0  Capacitance=1.0  Setx0=off  InitialVoltage=0  Measurements=Branch current
      settings: SourceProductBaseCode=MT,PS
  Switch1 : Switch  Threshold=1
  Synchronous Machine pu Standard : powerlib/Machines/Synchronous Machine pu Standard  PresetModel=No  MechanicalLoad=Mechanical power Pm  ShowDetailedParameters=on  RotorType=Salient-pole  Units=per unit standard parameters  MeasurementBus=off  NominalParameters="[ Pnom  Vnom_gen Fnom ]"  Reactances1=[ 1.81, 0.3, 0.23, 1.76, 0.65, 0.25, 0.15 ]  Reactances2="[ Xd, Xd1, Xd2, Xq,  Xq2,  Xl ]"  dAxisTimeConstants=Open-circuit  qAxisTimeConstants=Short-circuit  TimeConstants1="[ 4.4849  0.0681  0.1  ]"  TimeConstants2=[ 8.0, 0.03, 1.0, 0.07 ]  TimeConstants3="[  Tdo1  Tdo2  Tq2  ]"  TimeConstants4=[ 8.0, 0.03, 0.3371, 0.0295 ]  TimeConstants5=[ 1.01, 0.053, 0.1 ]  TimeConstants6=[ 1.3201, 0.023, 1.0, 0.07 ]  TimeConstants7="[  1.01  0.053  0.051266  ]"  TimeConstants8=[ 1.3201, 0.0231, 0.3371, 0.0295 ]  StatorResistance=Resistance  Mechanical=[ H F p]  PolePairs=1  InitialConditions=init  SetSaturation=off  Saturation=[0.6404,0.7127,0.8441,0.9214,0.9956,1.082,1.19,1.316,1.457;0.7,0.7698,0.8872,0.9466,0.9969,1.046,1.1,1.151,1.201]  LoadFlowParameters=[1,0,0,0,0]  TsPowergui=0  TsBlock=-1  IterativeModel=Trapezoidal non iterative  IterativeDiscreteModel=Trapezoidal non iterative  BusType=PV  Pref=0  Qref=0  Qmin=-inf  Qmax=inf  PLF=0  QLF=0
      settings: SourceProductBaseCode=MT,PS
  Terminator1 : Terminator
  Terminator2 : Terminator  Commented=on
  Terminator3 : Terminator  Commented=on
  Three-Phase Breaker : powerlib/Elements/Three-Phase Breaker  InitialState=closed  SwitchA=on  SwitchB=on  SwitchC=on  SwitchTimes=[1000]  External=on  BreakerResistance=Ron_breaker/Nb_WT  SnubberResistance=Rs_breaker/Nb_WT  SnubberCapacitance=Cs_breaker*Nb_WT  Measurements=None
  Universal Bridge : powerlib/Power Electronics/Universal Bridge  Arms=3  SnubberResistance=2*Ts_snub/(Pnom/(1000*2*pi*Fnom*Vnom_gen^2))  SnubberCapacitance=Pnom/(1000*2*pi*Fnom*Vnom_gen^2)  Device=Diodes  Ron=1e-6/Nb_wt  Lon=0  ForwardVoltages="[  0  0  ]"  ForwardVoltage=0  GTOparameters=[ 10e-6 , 20e-6 ]  IGBTparameters=[ 1e-6 , 2e-6 ]  Measurements=None  Measurements_2=None  converterType=Rectifier
      settings: SourceProductBaseCode=MT,PS
  V_ab : powerlib/Electrical Sources/Controlled Voltage Source  Initialize=on  Source_Type=AC  Amplitude=0  Phase=0  Frequency=0  Measurements=None
      settings: SourceProductBaseCode=MT,PS
  V_bc : powerlib/Electrical Sources/Controlled Voltage Source  Initialize=on  Source_Type=AC  Amplitude=0  Phase=0  Frequency=0  Measurements=None
      settings: SourceProductBaseCode=MT,PS
  Wind Turbine1 : Subsystem  mask(Wind Turbine){Prated=Pmec, c1_c8=c1_c8, K1_K2=K1_K2, wind0=wind0, Ts=Ts}
      mask prompts: Prated "Nominal mechanical output power (W):"; c1_c8 "Coefficients [c1 ... c8]"; K1_K2 "Parameters [K1 K2]"; wind0 "Initial wind speed (m/s):"; Ts "Sample time (s):"
      mask help:
      | This block implements a generic wind turbine models.
      |
      | The first input is the turbine speed in per unit of the generator base speed. For a synchronous or asynchronous generator, the base speed is the synchronous speed. For a permanent-magnet generator, the base speed is defined as the speed producing nominal voltage at  no load. The second input is the blade pitch angle in degrees. The third input is the wind speed in m/s.
      |
      | The output is the torque applied to the drive train in per unit based on the nominal power of the turbine and the base speed of the generator.
      mask init:
      | c1 = c1_c8(1);
      | c2 = c1_c8(2);
      | c3 = c1_c8(3);
      | c4 = c1_c8(4);
      | c5 = c1_c8(5);
      | c6 = c1_c8(6);
      | c7 = c1_c8(7);;
      | c8 = c1_c8(8);
      | 
      | K1=K1_K2(1);
      | K2=K1_K2(2);
      settings: OpenFcn=power_openblockproxy();
      mask Display: disp('');
  deg->rd : Gain  Gain=pi/180  SaturateOnIntegerOverflow=on  OutDataTypeStr=Inherit: Same as input  ParamDataTypeStr=Inherit: Same as input
  A : PMIOPort  Tag=PMCPort  Side=Left
  B : PMIOPort  Tag=PMCPort  Port=2  Side=Left
  C : PMIOPort  Tag=PMCPort  Port=3  Side=Left
  m : Outport  VectorParamsAs1DForOutWhenUnconnected=off
  tag scope: switch_WT=global
  wires:
  Bus Selector/2 -> deg->rd/1  "<Rotor mechanical angle  theta (deg)>"
  deg->rd/1 -> [angle_rotor]
  Bus Selector/1 -> [wr]  "<Rotor speed  wm  (pu)>"
  [Iabc_grid] -> Inverter and DC-DC Converter Average Models/2(Iabc_grid_conv)
  [IL] -> Inverter and DC-DC Converter Average Models/1(IL)
  [Vabc_grid] -> Control/1(Vabc_grid)
  [Iabc_grid] -> Control/2(Iabc_grid_conv)
  [Vabc_LL_stator] -> Control/3(Vabc_LL_stator)
  [Iabc_stator] -> Control/4(Iabc_stator)
  [Vdc] -> Control/6(Vdc)
  [angle_rotor] -> Control/7(angle_rotor)
  [wr] -> Control/8(wr)
  Control/2(Duty_Cycle) -> Inverter and DC-DC Converter Average Models/4(Duty_Cycle)  "Duty_cycle"
  Control/3(Pitch_angle) -> [Pitch]
  Control/4(Vf) -> [Vf]
  Control/5(PQ_pu) -> [PQ_pu]
  [IL] -> Control/5(IL)
  Control/1(U_ctrl_inverter) -> Inverter and DC-DC Converter Average Models/3(Uctrl_inverter)
  Inverter and DC-DC Converter Average Models/4(Vdc (V)) -> [Vdc]
  [Qcmd] -> Control/9(Qref)
  [Pitch] -> Wind Turbine1/2(Pitch angle (deg))
  Drive Train/2(T_shaft (pu)) -> Power base for the Generator/1
  Drive Train/1(W_wt (pu)) -> Wind Turbine1/1(W_wt (pu))
  "Wind (m/s) "/1 -> Wind Turbine1/3(Wind speed (m/s)), [U]
  Power base for the Generator/1 -> [Tm]
  [wr] -> Drive Train/2(Generator speed (pu))
  Wind Turbine1/1(Tt (pu)) -> Drive Train/1(T_wt (pu))
  Bus Selector/4 -> [Te]  "<Electromagnetic torque  Te (pu)>"
  Bus Selector/3 -> [Pe]  "<Electrical power  Pe (pu)>"
  Inverter and DC-DC Converter Average Models/1(Vab (V)) -> V_ab/1, [vab]
  [wr] -> Product/1
  B_gen/2 -> [Iabc_stator]
  Inverter and DC-DC Converter Average Models/2(Vbc (V)) -> V_bc/1, [vbc]
  B_switch/2 -> [Iabc_grid_i]
  Synchronous Machine pu Standard/1 -> Bus Selector/1
  B_switch/1 -> [Vabc_grid_i]
  [Tm] -> Product/2
  IL/1 -> -> pu/1
  B_gen/1 -> [Vabc_LL_stator]
  [Vf] -> Synchronous Machine pu Standard/2
  Inverter and DC-DC Converter Average Models/3(Vswitch (V)) -> Average Switch Voltage/1(Vswitch), [Vswitch]
  B_grid_conv/1 -> [Vabc_grid_conv]
  Product/1 -> Synchronous Machine pu Standard/1, [Pm_gen]
  -> pu/1 -> [IL]
  Control/6(protection) -> [protection]
  "Fault Controller (atomic) "/1(savgP) -> Goto18/1
  From35/1 -> "Fault Controller (atomic) "/1(Inport)
  "Fault Controller (atomic) "/8(Ppredict) -> Goto31/1
  "Fault Controller (atomic) "/2(genTemp) -> Goto19/1
  "Fault Controller (atomic) "/7(dTemp) -> Goto17/1
  "Fault Controller (atomic) "/6(Timers) -> Goto30/1
  "Fault Controller (atomic) "/3(dwHSS) -> Goto20/1
  "Fault Controller (atomic) "/5(mode) -> Goto23/1
  Gain8/1 -> Scope6/1  "Te/Tm"
  From80/1 -> Gain14/1
  From77/1 -> Demux2/1
  [Tm] -> Mux1/2
  From75/1 -> Mux10/2  "Qcmd"
  Mux12/1 -> Scope7/2
  From74/1 -> Mux8/1  "Pcmd"
  [Te] -> Mux1/1
  Mux9/1 -> Scope7/1
  Gain13/1 -> Mux15/3  "P"
  Gain14/1 -> Mux15/2  "Tm"
  Gain12/1 -> Mux12/2  "P"
  From70/1 -> Mux7/1  "Tgain"
  Gain9/1 -> Mux8/3  "P"
  [Pe] -> Mux4/2
  From82/1 -> Scope8/3  "wr"
  Demux1/1 -> Gain9/1
  Mux5/1 -> Scope13/2
  Mux4/1 -> Gain7/1  "Pe/Pm"
  From59/1 -> Scope8/1  "freq"
  Mux10/1 -> Scope9/3
  Demux1/2 -> Mux10/1  "Q"
  [Pm_gen] -> Mux4/1  "Pm"
  [Pitch] -> Scope6/4  "pitch"
  [PQ_pu] -> Gain2/1
  From73/1 -> Demux1/1
  Mux1/1 -> Gain8/1
  Mux8/1 -> Scope9/2
  Constant2/1 -> Mux9/3
  From78/1 -> Mux12/1  "Pcmd"
  Mux15/1 -> Scope8/2
  Gain11/1 -> Mux3/2  "P"
  Gain5/1 -> Mux7/2  "Tm"
  From72/1 -> Gain6/1  "Pm"
  [PQ_pu] -> Demux7/1
  From81/1 -> Mux15/1  "Tgain"
  Gain6/1 -> Mux8/2  "Pm"
  [Qcmd] -> Mux5/2  "Qcmd"
  From69/1 -> Gain5/1
  [wr] -> Scope6/3  "wr"
  Mux3/1 -> Scope13/1
  Demux2/1 -> Gain12/1
  Constant3/1 -> Mux9/2
  Constant5/1 -> Mux9/6
  Demux7/2 -> Mux5/1  "Q"
  From79/1 -> Demux3/1
  [Pcmd] -> Mux3/1  "Pcmd"
  Constant6/1 -> Mux9/4
  Demux3/1 -> Gain13/1
  Constant4/1 -> Mux9/5
  Gain2/1 -> Scope6/6  "PQ"
  Demux7/1 -> Gain11/1
  Mux7/1 -> Scope9/1
  From76/1 -> Mux9/1
  Gain7/1 -> Scope6/2  "Pe/Pm"
  [Pderate] -> Min1/2
  [Pcmd] -> Min1/1
  Min1/1 -> Control/10(Pcmd)
  [Pderate] -> Switch1/2
  Switch1/1 -> Control/11(Tgain)
  Constant1/1 -> Switch1/3
  [Tgain] -> Switch1/1
  PLL (3ph)2/2 -> Terminator1/1
  [Vabc_grid] -> PLL (3ph)2/1
  PLL (3ph)2/1 -> [f_grid]  "f(wind)"
  [Qin] -> APC (atomic)1/6(Qin)
  [f_grid] -> APC (atomic)1/1(Freq (Hz))
  APC (atomic)1/3(Qcmd) -> [Qcmd]
  APC (atomic)1/2(Tcmd) -> [Tgain]
  [protection] -> APC (atomic)1/7(protection)
  [wr] -> APC (atomic)1/3(wr [pu])
  APC (atomic)1/1(Pcmd) -> [Pcmd]
  [Pin] -> APC (atomic)1/4(Pin)
  [mode] -> Control/12(Mode)
  [Pm_gen] -> Bus Creator/8  "Pm_gen_pu"
  Bus Creator/1 -> m/1
  [Iabc_grid] -> Bus Creator/5  "Iabc_grid_conv_pu"
  [Pitch] -> Bus Creator/9  "Pitch_deg"
  [PQ_pu] -> Bus Creator/11  "PQ_pu"
  [Vf] -> Bus Creator/6  "Vfield_pu"
  [Vdc] -> Bus Creator/10  "Vdc_V"
  [Vabc_LL_stator] -> Bus Creator/1  "Vabc_stator_pu"
  [Vabc_grid] -> Bus Creator/3  "Vabc_grid_pu"
  [Iabc_stator] -> Bus Creator/2  "Iabc_stator_pu"
  [wr] -> Bus Creator/7  "wr_pu"
  [Vabc_grid_conv] -> Bus Creator/4  "Vabc_grid_conv_pu"
  B_grid/2 -> [Iabc_grid]
  B_grid/1 -> [Vabc_grid]
  PLL (3ph)1/1 -> Goto32/1
  PLL (3ph)1/2 -> Terminator2/1
  From30/1 -> PLL (3ph)1/1
  From31/1 -> Mux/1
  From33/1 -> Mux/2
  From34/1 -> Mux2/1
  From36/1 -> Mux2/2
  Mux2/1 -> Scope/2
  Mux/1 -> Scope/1
  From40/1 -> Scope2/1  "iabc stator"
  From41/1 -> Scope2/2  "vabs ll stator"
  From42/1 -> Scope2/3  "IL"
  From43/1 -> Scope2/4  "vabc grid conv"
  From45/1 -> Scope2/6  "Vdc"
  From46/1 -> Scope2/7  "Vswitch"
  From50/1 -> Scope2/8  "Vab"
  From57/1 -> Scope2/9  "Vbc"
  Sequence Analyzer/1 -> Mux11/1  "V(wind)"
  Constant13/1 -> Mux11/6
  Constant15/1 -> Mux11/5
  Constant14/1 -> Mux11/7
  Constant12/1 -> Mux11/3
  Constant11/1 -> Mux11/4
  Mux11/1 -> Scope3/1
  From66/1 -> Sequence Analyzer/1  "V"
  Constant16/1 -> Mux11/2
  Demux6/2 -> Scope3/2  "Q"
  From60/1 -> Demux6/1
  "Power (3ph, Phasor)2"/2 -> Mux13/2  "Q(Wind)"
  From63/1 -> "Power (3ph, Phasor)2"/1
  "Power (3ph, Phasor)2"/1 -> Mux13/1  "P(Wind)"
  From64/1 -> "Power (3ph, Phasor)2"/2
  Mux13/1 -> Scope4/1  "PQ_grid"
  Mux19/1 -> Scope4/2  "PQ_grid2"
  From71/1 -> "Power (3ph, Phasor)1"/2
  From67/1 -> "Power (3ph, Phasor)1"/1
  "Power (3ph, Phasor)1"/1 -> Mux19/1  "P(Wind)"
  "Power (3ph, Phasor)1"/2 -> Mux19/2  "Q(Wind)"
  PLL (3ph)3/1 -> Goto38/1
  PLL (3ph)3/2 -> Terminator3/1
  From98/1 -> PLL (3ph)3/1
  From99/1 -> Mux/3
  From87/1 -> Mux2/3
  From37/1 -> Mux6/1
  From38/1 -> Mux6/2
  From96/1 -> Mux6/3
  Mux6/1 -> Scope/3
  B_grid_conv/2 -> [Iabc_grid_conv]
  From100/1 -> Scope2/5
  Bus Selector1/3 -> Demux8/1  "<WT PQ cmd>"
  Demux8/1 -> [Pin]
  Demux8/2 -> [Qin]
  Bus Selector1/4 -> [f_setpoint]  "<f setpoint>"
  Bus Selector1/5 -> [V_setpoint]  "<V setpoint>"
  [switch_cmd] -> AND/1
  [protection] -> Scope1/1, AND/2
  AND/1 -> [switch_WT], Three-Phase Breaker/1
  [mode] -> APC (atomic)1/5(case)
  [f_setpoint] -> APC (atomic)1/2(f_setpoint)
  [V_setpoint] -> Control/13(V_setpoint)
  [MGCC_cmd] -> Bus Selector1/1
  Bus Selector1/1 -> [switch_cmd]  "<WT switch req>"
  Bus Selector1/2 -> [mode]  "<WT mode>"
  Constant/1 -> [Pderate]
  [U] -> 5-s avg/1
  5-s avg/1 -> Control/14(U5s)
  [U] -> Scope6/5  "U"
  connections:
  B_grid/RConn1 -- Three-Phase Breaker/RConn1
  B_grid/RConn2 -- Three-Phase Breaker/RConn2
  Three-Phase Breaker/RConn3 -- B_grid/RConn3
  B_grid_conv/RConn2 -- V_bc/RConn1 -- V_ab/LConn1
  Three-Phase Breaker/LConn3 -- B_switch/LConn3
  Three-Phase Breaker/LConn2 -- B_switch/LConn2
  B_switch/LConn1 -- Three-Phase Breaker/LConn1
  B_switch/RConn3 -- "Choke "/LConn3
  "Choke "/RConn3 -- B_grid_conv/LConn3
  B_switch/RConn2 -- "Choke "/LConn2
  Universal Bridge/LConn1 -- B_gen/LConn1
  B_gen/RConn2 -- Synchronous Machine pu Standard/RConn2
  Average Switch Voltage/RConn1 -- IL/RConn1
  Universal Bridge/LConn2 -- B_gen/LConn2
  Universal Bridge/LConn3 -- B_gen/LConn3
  V_ab/RConn1 -- B_grid_conv/RConn1
  B_switch/RConn1 -- "Choke "/LConn1
  B_gen/RConn1 -- Synchronous Machine pu Standard/RConn1
  "Choke "/RConn1 -- B_grid_conv/LConn1
  "Choke "/RConn2 -- B_grid_conv/LConn2
  B_grid_conv/RConn3 -- V_bc/LConn1
  Series RLC Branch1/LConn1 -- Universal Bridge/RConn1
  B_gen/RConn3 -- Synchronous Machine pu Standard/RConn3
  Series RLC Branch1/RConn1 -- IL/LConn1
  Average Switch Voltage/LConn1 -- Universal Bridge/RConn2
  A/RConn1 -- Filter Q=1/LConn1 -- B_grid/LConn1
  B/RConn1 -- Filter Q=1/LConn2 -- B_grid/LConn2
  C/RConn1 -- Filter Q=1/LConn3 -- B_grid/LConn3

== system Auto_microgrid_forecasting_020822/induction attempts2 ==
  Asynchronous Machine pu ABB 1.8MW : powerlib/Machines/Asynchronous Machine pu Units  Commented=on  RotorType=Squirrel-cage  PresetModel=No  MechanicalLoad=Torque Tm  ShowDetailedParameters=on  ReferenceFrame=Rotor  Units=pu  MeasurementBus=off  NominalParameters=[1.8e+06 1e+04 60]  Stator=[0.02565 0.09937]  Rotor=[0.01909 0.0397]  Cage1=[0.004672 0.11]  Cage2=[0.04455 0.09937]  Lm=3.275  Mechanical=[0.09526 0.05479 2]  PolePairs=2  InitialConditions="[ 0.01,0   0,0,0   0,0,0 ]"  SimulateSaturation=off  Saturation="[0.212,0.4201,0.8125,1.0979,1.4799,2.2457,3.2586,4.5763,6.4763 ;   0.5,0.7,0.9,1,1.1,1.2 ,1.3,1.4,1.5]"  LoadFlowParameters=0  TsPowergui=0  TsBlock=-1  IterativeModel=Trapezoidal non iterative  IterativeDiscreteModel=Trapezoidal non iterative  Pmec=0
      settings: SourceProductBaseCode=PS
  Asynchronous Machine pu Baldor 500HP : powerlib/Machines/Asynchronous Machine pu Units  RotorType=Squirrel-cage  PresetModel=No  MechanicalLoad=Torque Tm  ShowDetailedParameters=on  ReferenceFrame=Rotor  Units=pu  MeasurementBus=off  NominalParameters=[3.731e+05 460 60]  Stator=[0.02671 0.07843]  Rotor=[0.01909 0.0397]  Cage1=[0.00673 0.1222]  Cage2=[0.05602 0.07843]  Lm=3.861  Mechanical=[0.09526 0.05479 1]  PolePairs=2  InitialConditions="[ 0.01,0   0,0,0   0,0,0 ]"  SimulateSaturation=off  Saturation="[0.212,0.4201,0.8125,1.0979,1.4799,2.2457,3.2586,4.5763,6.4763 ;   0.5,0.7,0.9,1,1.1,1.2 ,1.3,1.4,1.5]"  LoadFlowParameters=0  TsPowergui=0  TsBlock=-1  IterativeModel=Trapezoidal non iterative  IterativeDiscreteModel=Trapezoidal non iterative  Pmec=0
      settings: SourceProductBaseCode=PS
  Asynchronous Machine pu FCgen : powerlib/Machines/Asynchronous Machine pu Units  Commented=on  RotorType=Squirrel-cage  PresetModel=No  MechanicalLoad=Torque Tm  ShowDetailedParameters=on  ReferenceFrame=Rotor  Units=pu  MeasurementBus=off  NominalParameters=[2.02e+06 460 60]  Stator=[-0.005 0.09337]  Rotor=[0.01909 0.0397]  Cage1=[-0.01 0.2054]  Cage2=[-0.06 0.09337]  Lm=1.867  Mechanical=[0.09526 0.05479 1]  PolePairs=2  InitialConditions="[ 0.01, 0,   0,0,0   0,0,0 ]"  SimulateSaturation=off  Saturation="[0.212,0.4201,0.8125,1.0979,1.4799,2.2457,3.2586,4.5763,6.4763 ;   0.5,0.7,0.9,1,1.1,1.2 ,1.3,1.4,1.5]"  LoadFlowParameters=0  TsPowergui=0  TsBlock=Ts  IterativeModel=Trapezoidal non iterative  IterativeDiscreteModel=Trapezoidal non iterative  Pmec=0
      settings: SourceProductBaseCode=PS
  Bus Selector : BusSelector  OutputSignals=Mechanical.Electromagnetic torque Te (pu),Mechanical.Rotor speed (wm)
  Bus Selector2 : BusSelector  OutputSignals=Mechanical.Rotor speed (wm)  OutputAsBus=on
  Diesel Engine Governor : spsDieselMotorModel/Diesel Engine Governor  K=10/4  Tr=[0.01 0.02 0.2]  Ta=[0.2 0.009 0.0384]  Tlim=[0 1.1]  Td=0.05  Pm0=0.126/0.126
      settings: SourceProductBaseCode=PS
  Divide : Product  Inputs=*/
  Divide1 : Product  Inputs=**
  Gain1 : Gain  Gain=1.8e6
  SM 3.125 MVA1 : powerlib/Machines/Synchronous Machine pu Standard  Commented=on  PresetModel=No  MechanicalLoad=Mechanical power Pm  ShowDetailedParameters=on  RotorType=Salient-pole  Units=per unit standard parameters  MeasurementBus=off  NominalParameters=[2e+06 460 60]  Reactances1=[ 31 32 33 34 35 36 37 ]  Reactances2=[3.08 0.24 0.18 2.28 0.23 0.04]  dAxisTimeConstants=Short-circuit  qAxisTimeConstants=Short-circuit  TimeConstants1=[]  TimeConstants2=[]  TimeConstants3=[]  TimeConstants4=[]  TimeConstants5=[ 3.7, 0.05, 0.05 ]  TimeConstants6=[ 8.0, 0.03, 0.3371, 0.0295 ]  TimeConstants7=[0.29 0.03 0.03]  TimeConstants8=[]  StatorResistance=0.012007561436673  Mechanical=[1 0.01231 2]  PolePairs=2  InitialConditions=[0 0 0 0 0 0 0 0 1]  SetSaturation=off  Saturation=[0.211 0.418 1.0 1.25 1.72 3.35 ;0.25 0.50 1.0 1.1 1.2 1.4]  LoadFlowParameters=[1 0 0 0]  TsPowergui=0  TsBlock=Ts  IterativeModel=Trapezoidal non iterative  IterativeDiscreteModel=Backward Euler robust  BusType=PV  Pref=0  Qref=0  Qmin=-Inf  Qmax=Inf  PLF=0  QLF=0
      settings: AttributesFormatString=\n\n  SourceProductBaseCode=MT,PS
  Scope : Scope  NumInputPorts=3
  Scope1 : Scope  NumInputPorts=3
  Scope2 : Scope
  wref (pu) : Constant
  A : PMIOPort  Side=Right
  B : PMIOPort  Port=2  Side=Right
  C : PMIOPort  Port=3  Side=Right
  wires:
  Asynchronous Machine pu Baldor 500HP/1 -> Bus Selector/1, Bus Selector2/1
  Diesel Engine Governor/1 -> Scope1/1, Divide/1  "Pm"
  wref (pu)/1 -> Diesel Engine Governor/1
  Bus Selector2/1 -> Scope1/3, Divide/2, Diesel Engine Governor/2  "Wm"
  Divide/1 -> Asynchronous Machine pu Baldor 500HP/1, Scope1/2
  Bus Selector/1 -> Scope/2, Divide1/1  "<Electromagnetic torque Te (pu)>"
  Bus Selector/2 -> Scope/1, Divide1/2  "<Rotor speed (wm)>"
  Divide1/1 -> Gain1/1, Scope/3
  Gain1/1 -> Scope2/1
  connections:
  Asynchronous Machine pu Baldor 500HP/LConn3 -- C/RConn1
  Asynchronous Machine pu Baldor 500HP/LConn1 -- A/RConn1
  Asynchronous Machine pu Baldor 500HP/LConn2 -- B/RConn1

== system Auto_microgrid_forecasting_020822/synchronous ==
  note: try adding a delay to Vf
  Bus Selector : BusSelector  OutputSignals="Output active power   Peo (pu),Output reactive power  Qeo (pu),Mechanical.Electrical power  Pe (pu)"
  Bus Selector1 : BusSelector  OutputSignals=f setpoint,V setpoint
  Bus Selector2 : BusSelector  OutputSignals="Mechanical.Rotor speed  wm  (pu)"  OutputAsBus=on
  Bus Selector4 : BusSelector  OutputSignals="dq0 components.Field current  ifd (pu)"  OutputAsBus=on
  Bus Selector5 : BusSelector  OutputSignals="dq0 components.Stator voltage  vd (pu),dq0 components.Stator voltage  vq (pu)"  OutputAsBus=on
  Bus Selector6 : BusSelector  OutputSignals="dq0 components.Stator current  id (pu),dq0 components.Stator current  iq (pu)"  OutputAsBus=on
  Delay : Delay  DelayLength=0
  Diesel Engine Governor : spsDieselMotorModel/Diesel Engine Governor  K=10  Tr=[0.01 0.02 0.2]  Ta=[0.2 0.009 0.0384]  Tlim=[0 1.1]  Td=0.05  Pm0=0.126
      settings: SourceProductBaseCode=PS
  EXCITATION : Subsystem  Variant=on  VariantControlMode=Label  LabelModeActiveChoice=Variant1
      settings: AttributesFormatString=%<BlockChoice>
  Fcn1 : Fcn  Expr=sqrt(u(1)^2 + u(2)^2)
  Fcn2 : Fcn  Expr=sqrt(u(1)^2 + u(2)^2)
  Ground : Ground
  SM : Scope  NumInputPorts=4
  SM 3.125 MVA : powerlib/Machines/Synchronous Machine pu Standard  PresetModel=No  MechanicalLoad=Mechanical power Pm  ShowDetailedParameters=on  RotorType=Salient-pole  Units=per unit standard parameters  MeasurementBus=off  NominalParameters=[2e+06 460 60]  Reactances1=[ 31 32 33 34 35 36 37 ]  Reactances2=[3.08 0.24 0.18 2.28 0.23 0.04]  dAxisTimeConstants=Short-circuit  qAxisTimeConstants=Short-circuit  TimeConstants1=[]  TimeConstants2=[]  TimeConstants3=[]  TimeConstants4=[]  TimeConstants5=[ 3.7, 0.05, 0.05 ]  TimeConstants6=[ 8.0, 0.03, 0.3371, 0.0295 ]  TimeConstants7=[0.29 0.03 0.03]  TimeConstants8=[]  StatorResistance=0.012007561436673  Mechanical=[1 0.01231 2]  PolePairs=2  InitialConditions=[0 0 0 0 0 0 0 0 1]  SetSaturation=off  Saturation=[0.211 0.418 1.0 1.25 1.72 3.35 ;0.25 0.50 1.0 1.1 1.2 1.4]  LoadFlowParameters=[1 0 0 0]  TsPowergui=0  TsBlock=Ts  IterativeModel=Trapezoidal non iterative  IterativeDiscreteModel=Backward Euler robust  BusType=PV  Pref=0  Qref=0  Qmin=-Inf  Qmax=Inf  PLF=0  QLF=0
      settings: AttributesFormatString=\n\n  SourceProductBaseCode=MT,PS
  Scope : Scope  NumInputPorts=3
  Scope1 : Scope
  A : PMIOPort  Side=Right
  B : PMIOPort  Port=2  Side=Right
  C : PMIOPort  Port=3  Side=Right
  wires:
  Bus Selector1/1 -> Diesel Engine Governor/1, Scope1/1  "<f setpoint>"
  Bus Selector5/1 -> Fcn1/1  "Vd Vq"
  SM 3.125 MVA/1 -> Bus Selector/1, Bus Selector2/1, Bus Selector4/1, Bus Selector6/1, Bus Selector5/1
  Fcn2/1 -> EXCITATION/3(It)
  Bus Selector1/2 -> EXCITATION/1(Vref)  "<V setpoint>"
  Bus Selector6/1 -> Fcn2/1  "Id Iq"
  EXCITATION/1(Efd) -> Delay/1  "Vf"
  Bus Selector4/1 -> EXCITATION/4(Ifd)  "Ifd"
  Diesel Engine Governor/1 -> SM/3, SM 3.125 MVA/1  "Pm"
  Ground/1 -> EXCITATION/5(Vstab)  "Not implemented"
  Fcn1/1 -> EXCITATION/2(Vt)  "Vt"
  Bus Selector2/1 -> SM/1, Diesel Engine Governor/2  "w"
  Bus Selector/1 -> SM/2, Scope/1  "<Output active power   Peo (pu)>"
  Bus Selector/2 -> Scope/2  "<Output reactive power  Qeo (pu)>"
  Bus Selector/3 -> Scope/3  "<Electrical power  Pe (pu)>"
  Delay/1 -> SM 3.125 MVA/2, SM/4  "Vf"
  [MGCC_cmd] -> Bus Selector1/1
  connections:
  SM 3.125 MVA/RConn3 -- C/RConn1
  SM 3.125 MVA/RConn1 -- A/RConn1
  SM 3.125 MVA/RConn2 -- B/RConn1
